simulink model "model1_unstable_controller_observer"  (R2022b)
settings: Solver=VariableStepAuto  StartTime=0.0  StopTime=10.0  RelTol=1e-3
InitFcn:
  | model1_init_params_unstable
  | % model1_init_params_stable
values from neighbouring files (symbols this model uses):
  a = 0.347    [model1_init_params_stable.m]    (also in model1_init_params_unstable.m)
  A = [ ... (first row only)    [model1_init_params_stable.m]    (also in model1_init_params_unstable.m; model2_init_params_stable.m; model2_init_params_unstable.m; model2_init_params_unstable__lqr_controller.m)
  A_obs = A-L*C    [model1_init_params_stable.m]    (also in model1_init_params_unstable.m; model2_init_params_unstable__lqr_controller.m = A_ccf-L*C_ccf)
  b = 1.02    [model1_init_params_stable.m]    (also in model1_init_params_unstable.m)
  B = [ ... (first row only)    [model1_init_params_stable.m]    (also in model1_init_params_unstable.m; model2_init_params_stable.m; model2_init_params_unstable.m; model2_init_params_unstable__lqr_controller.m)
  B_obs = [B L]    [model1_init_params_stable.m]    (also in model1_init_params_unstable.m; model2_init_params_unstable__lqr_controller.m = [B_ccf L])
  c = 0.08    [model1_init_params_stable.m]    (also in model1_init_params_unstable.m)
  C = [(V^2*h-a*c*g)*sin(lambda)/(b*h^2)*k1 a*V*sin(lambda)/(b*h)*k1]    [model1_init_params_stable.m]    (also in model1_init_params_unstable.m; model2_init_params_stable.m = [1 0 0 0]; model2_init_params_unstable.m = [1 0 0 0]; model2_init_params_unstable__lqr_controller.m = [1 0 0 0])
  C_obs = eye(length(A_obs))    [model1_init_params_stable.m]    (also in model1_init_params_unstable.m; model2_init_params_unstable__lqr_controller.m)
  D = 0    [model1_init_params_stable.m]    (also in model1_init_params_unstable.m; model2_init_params_stable.m; model2_init_params_unstable.m; model2_init_params_unstable__lqr_controller.m)
  D_obs = zeros(size(B_obs))    [model1_init_params_stable.m]    (also in model1_init_params_unstable.m; model2_init_params_unstable__lqr_controller.m)
  g = 9.81    [model1_init_params_stable.m]    (also in model1_init_params_unstable.m)
  h = 0.8603    [model1_init_params_stable.m]    (also in model1_init_params_unstable.m)
  K = place(A,B,new_poles)    [model1_init_params_unstable.m]    (also in model2_init_params_unstable.m = place(A_ccf,B_ccf,new_poles))
  k1 = b^2/((V^2*sin(lambda) - b*g*cos(lambda))*m*a*c*sin(lambda))    [model1_init_params_stable.m]    (also in model1_init_params_unstable.m)
  k2 = b*g/(V^2*sin(lambda) - b*g*cos(lambda))    [model1_init_params_stable.m]    (also in model1_init_params_unstable.m)
  lambda = pi/10    (= 0.314159265359)    [model1_init_params_stable.m]    (also in model1_init_params_unstable.m)
  V = 5.7    [model1_init_params_stable.m]    (also in model1_init_params_unstable.m = 3; model2_init_params_stable.m = 6.1; model2_init_params_unstable.m = 5; model2_init_params_unstable__lqr_controller.m = 5)
settings Model: Creator=neotod  LastModifiedBy=neotod

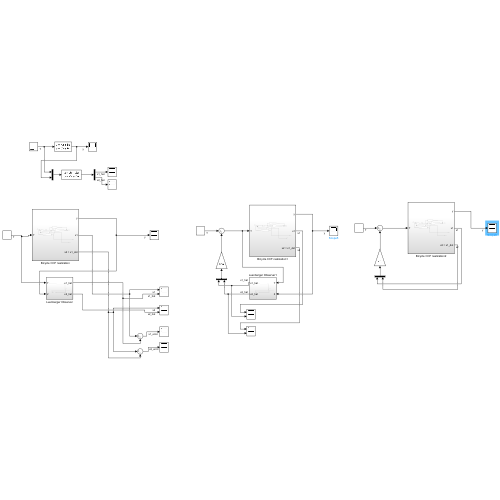
[thumbnail: Simulink's stored preview of the top-level diagram]
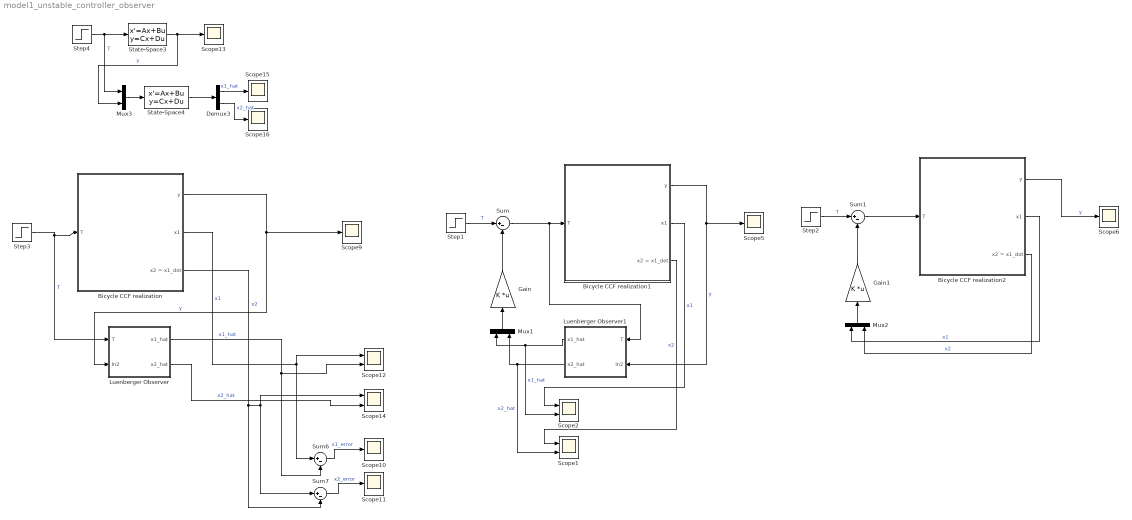
== system model1_unstable_controller_observer ==
  Bicycle CCF realization : Subsystem
  Bicycle CCF realization1 : Subsystem
  Bicycle CCF realization2 : Subsystem
  Demux3 : Demux  Outputs=2
  Gain : Gain  Gain=K  Multiplication=Matrix(K*u)
  Gain1 : Gain  Gain=K  Multiplication=Matrix(K*u)
  Luenberger Observer : Subsystem
  Luenberger Observer1 : Subsystem
  Mux1 : Mux  Inputs=2
  Mux2 : Mux  Inputs=2
  Mux3 : Mux  Inputs=2
  Scope{1..2,12,14} (4 alike) : Scope  NumInputPorts=2
  Scope{5..6,9..11,13,15..16} (8 alike) : Scope
  State-Space3 : StateSpace  A=A  B=B  C=C  D=D  InitialCondition=0
  State-Space4 : StateSpace  A=A_obs  B=B_obs  C=C_obs  D=D_obs  InitialCondition=0
  Step{1..4} (4 alike) : Step  SampleTime=0
  Sum{,1,6..7} (4 alike) : Sum  Inputs=|+-
  wires:
  Step3/1 -> Luenberger Observer/1(T), Bicycle CCF realization/1(T)  "T"
  Step4/1 -> Mux3/1, State-Space3/1  "T"
  State-Space3/1 -> Mux3/2, Scope13/1  "y"
  State-Space4/1 -> Demux3/1
  Mux3/1 -> State-Space4/1
  Demux3/1 -> Scope15/1  "x1_hat"
  Demux3/2 -> Scope16/1  "x2_hat"
  Sum6/1 -> Scope10/1  "x1_error"
  Sum7/1 -> Scope11/1  "x2_error"
  Bicycle CCF realization/2(x1) -> Sum6/1, Scope12/1  "x1"
  Bicycle CCF realization/1(y) -> Luenberger Observer/2(In2), Scope9/1  "y"
  Bicycle CCF realization/3(x2 = x1_dot) -> Sum7/2, Sum7/1, Scope14/1  "x2"
  Luenberger Observer/1(x1_hat) -> Sum6/2, Scope12/2  "x1_hat"
  Luenberger Observer/2(x2_hat) -> Scope14/2  "x2_hat"
  Bicycle CCF realization1/1(y) -> Luenberger Observer1/2(In2), Scope5/1  "y"
  Step1/1 -> Sum/1  "T"
  Sum/1 -> Luenberger Observer1/1(T), Bicycle CCF realization1/1(T)
  Gain/1 -> Sum/2
  Mux1/1 -> Gain/1
  Luenberger Observer1/1(x1_hat) -> Scope2/2, Mux1/1  "x1_hat"
  Luenberger Observer1/2(x2_hat) -> Scope1/2, Mux1/2  "x2_hat"
  Bicycle CCF realization1/2(x1) -> Scope2/1  "x1"
  Bicycle CCF realization1/3(x2 = x1_dot) -> Scope1/1  "x2"
  Sum1/1 -> Bicycle CCF realization2/1(T)
  Mux2/1 -> Gain1/1
  Step2/1 -> Sum1/1  "T"
  Gain1/1 -> Sum1/2
  Bicycle CCF realization2/1(y) -> Scope6/1  "y"
  Bicycle CCF realization2/2(x1) -> Mux2/1  "x1"
  Bicycle CCF realization2/3(x2 = x1_dot) -> Mux2/2  "x2"

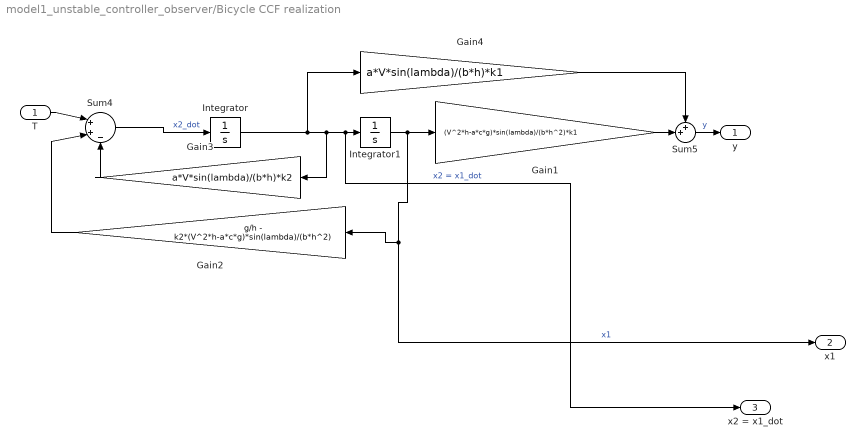
== system model1_unstable_controller_observer/Bicycle CCF realization ==
  T : Inport
  Gain1 : Gain  Gain=(V^2*h-a*c*g)*sin(lambda)/(b*h^2)*k1
  Gain2 : Gain  Gain=g/h - k2*(V^2*h-a*c*g)*sin(lambda)/(b*h^2)
  Gain3 : Gain  Gain=a*V*sin(lambda)/(b*h)*k2
  Gain4 : Gain  Gain=a*V*sin(lambda)/(b*h)*k1
  Integrator : Integrator
  Integrator1 : Integrator
  Sum4 : Sum  Inputs=|++-
  Sum5 : Sum  Inputs=++|
  y : Outport
  x1 : Outport  Port=2
  x2 = x1_dot : Outport  Port=3
  wires:
  Integrator/1 -> Gain4/1, Gain3/1, x2 = x1_dot/1, Integrator1/1  "x2 = x1_dot"
  Gain4/1 -> Sum5/1
  Gain2/1 -> Sum4/2
  Integrator1/1 -> Gain1/1, x1/1, Gain2/1  "x1"
  T/1 -> Sum4/1
  Sum4/1 -> Integrator/1  "x2_dot"
  Gain3/1 -> Sum4/3
  Gain1/1 -> Sum5/2
  Sum5/1 -> y/1  "y"

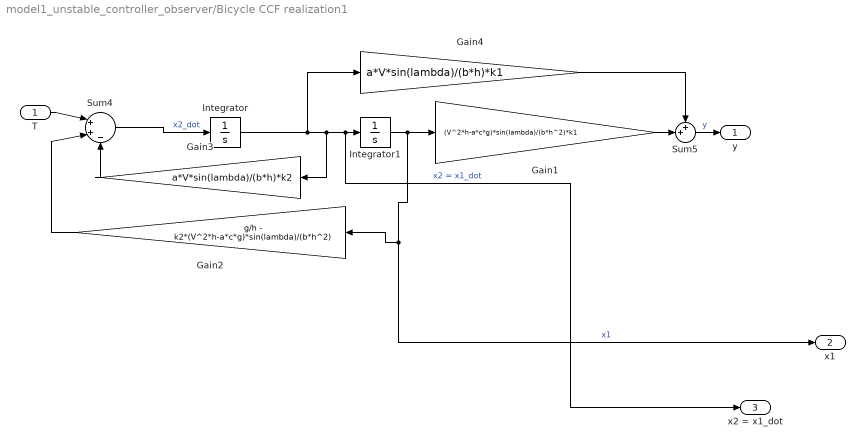
== system model1_unstable_controller_observer/Bicycle CCF realization1 ==
  T : Inport
  Gain1 : Gain  Gain=(V^2*h-a*c*g)*sin(lambda)/(b*h^2)*k1
  Gain2 : Gain  Gain=g/h - k2*(V^2*h-a*c*g)*sin(lambda)/(b*h^2)
  Gain3 : Gain  Gain=a*V*sin(lambda)/(b*h)*k2
  Gain4 : Gain  Gain=a*V*sin(lambda)/(b*h)*k1
  Integrator : Integrator
  Integrator1 : Integrator
  Sum4 : Sum  Inputs=|++-
  Sum5 : Sum  Inputs=++|
  y : Outport
  x1 : Outport  Port=2
  x2 = x1_dot : Outport  Port=3
  wires:
  Integrator/1 -> Gain4/1, Gain3/1, x2 = x1_dot/1, Integrator1/1  "x2 = x1_dot"
  Gain4/1 -> Sum5/1
  Gain2/1 -> Sum4/2
  Integrator1/1 -> Gain1/1, x1/1, Gain2/1  "x1"
  T/1 -> Sum4/1
  Sum4/1 -> Integrator/1  "x2_dot"
  Gain3/1 -> Sum4/3
  Gain1/1 -> Sum5/2
  Sum5/1 -> y/1  "y"

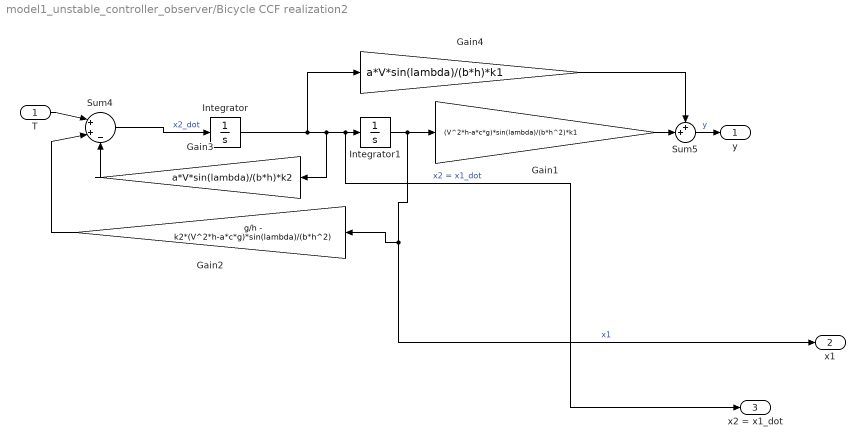
== system model1_unstable_controller_observer/Bicycle CCF realization2 ==
  T : Inport
  Gain1 : Gain  Gain=(V^2*h-a*c*g)*sin(lambda)/(b*h^2)*k1
  Gain2 : Gain  Gain=g/h - k2*(V^2*h-a*c*g)*sin(lambda)/(b*h^2)
  Gain3 : Gain  Gain=a*V*sin(lambda)/(b*h)*k2
  Gain4 : Gain  Gain=a*V*sin(lambda)/(b*h)*k1
  Integrator : Integrator
  Integrator1 : Integrator
  Sum4 : Sum  Inputs=|++-
  Sum5 : Sum  Inputs=++|
  y : Outport
  x1 : Outport  Port=2
  x2 = x1_dot : Outport  Port=3
  wires:
  Integrator/1 -> Gain4/1, Gain3/1, x2 = x1_dot/1, Integrator1/1  "x2 = x1_dot"
  Gain4/1 -> Sum5/1
  Gain2/1 -> Sum4/2
  Integrator1/1 -> Gain1/1, x1/1, Gain2/1  "x1"
  T/1 -> Sum4/1
  Sum4/1 -> Integrator/1  "x2_dot"
  Gain3/1 -> Sum4/3
  Gain1/1 -> Sum5/2
  Sum5/1 -> y/1  "y"

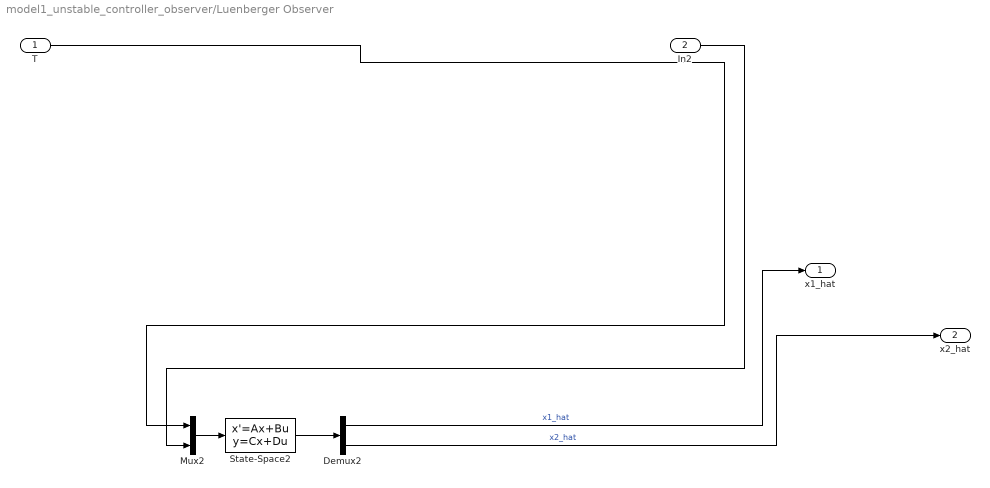
== system model1_unstable_controller_observer/Luenberger Observer ==
  T : Inport
  In2 : Inport  Port=2
  Demux2 : Demux  Outputs=2
  Mux2 : Mux  Inputs=2
  State-Space2 : StateSpace  A=A_obs  B=B_obs  C=C_obs  D=D_obs  InitialCondition=0
  x1_hat : Outport
  x2_hat : Outport  Port=2
  wires:
  Mux2/1 -> State-Space2/1
  In2/1 -> Mux2/2
  State-Space2/1 -> Demux2/1
  Demux2/2 -> x2_hat/1  "x2_hat"
  Demux2/1 -> x1_hat/1  "x1_hat"
  T/1 -> Mux2/1

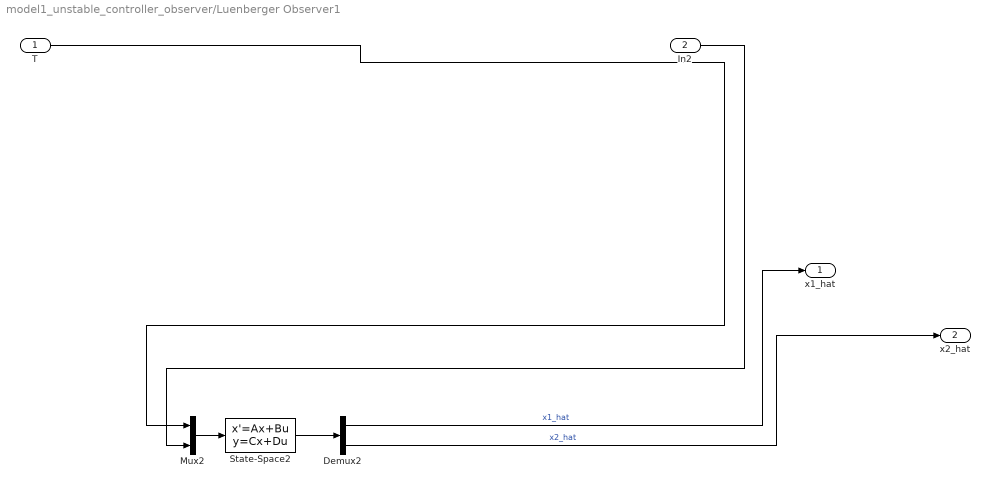
== system model1_unstable_controller_observer/Luenberger Observer1 ==
  T : Inport
  In2 : Inport  Port=2
  Demux2 : Demux  Outputs=2
  Mux2 : Mux  Inputs=2
  State-Space2 : StateSpace  A=A_obs  B=B_obs  C=C_obs  D=D_obs  InitialCondition=0
  x1_hat : Outport
  x2_hat : Outport  Port=2
  wires:
  Mux2/1 -> State-Space2/1
  In2/1 -> Mux2/2
  State-Space2/1 -> Demux2/1
  Demux2/2 -> x2_hat/1  "x2_hat"
  Demux2/1 -> x1_hat/1  "x1_hat"
  T/1 -> Mux2/1
